simulink model "ModelMy"  (R2023a)
settings: Solver=VariableStepAuto  StartTime=0.0  StopTime=0.01  FixedStep=1E-9  MaxStep=1E-9  RelTol=1e-5
libraries: spsDiodeLib x8, spsSeriesRLCBranchLib x8, spsIdealSwitchLib x4, simulink x3, spsVoltageMeasurementLib x3, spsDCVoltageSourceLib x1, spsGroundLib x1, spsLinearTransformerLib x1, spsMultimeterLib x1, simulink_extras x1, spspowerguiLib x1
settings Model: Creator=kva  LastModifiedBy=User
settings SolverCC: AlgebraicLoopSolver=TrustRegion
settings DataIOCC: ReturnWorkspaceOutputs=off
settings DebuggingCC: UnconnectedInputMsg=warning  UnconnectedOutputMsg=warning  UnconnectedLineMsg=warning  ArithmeticOperatorsInVariantConditions=warning
settings ModelReferenceCC: EnableRefExpFcnMdlSchedulingChecks=on
settings SFSimCC: CustomCodeUndefinedFunction=UseInterfaceOnly

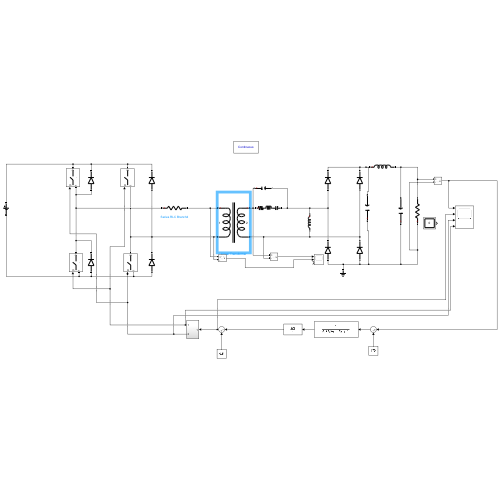
[thumbnail: Simulink's stored preview of the top-level diagram]
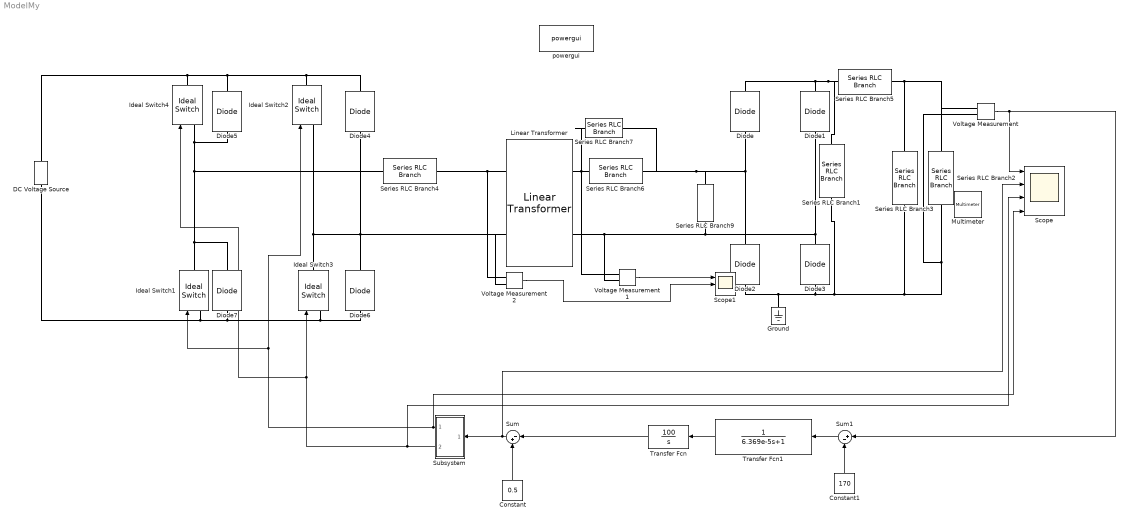
== system ModelMy ==
  Constant : Constant  Value=0.5
  Constant1 : Constant  Value=170
  DC Voltage Source : spsDCVoltageSourceLib/DC Voltage Source  Amplitude=42  Measurements=Voltage
  Diode{,1..7} (8 alike) : spsDiodeLib/Diode  Ron=0.001  Lon=0  Vf=1  IC=0  UseSnubber=0  Rs=inf  Cs=250e-9  Measurements=off
  Ground : spsGroundLib/Ground  LConnTagsString=a
  Ideal Switch{1..4} (4 alike) : spsIdealSwitchLib/Ideal Switch  Ron=0.001  Lon=0  IC=1  Rs=inf  Cs=inf  Measurements=off
  Linear Transformer : spsLinearTransformerLib/Linear Transformer  UNITS=SI  NominalPower=[ 250e6 60 ]  winding1=[42 0 0]  winding2=[170 0 0]  ThreeWindings=off  winding3=[3.15e+05 0.7938 0.084225]  RmLm=[Inf Inf]  Measurements=None  DataType=on
  Multimeter : spsMultimeterLib/Multimeter  L=2  sel=1  yselected={}  Gain=0  OutputType=Complex  PlotAtSimulationStop=off  PhasorSimulation=off
  Scope : Scope  NumInputPorts=4
  Scope1 : Scope  NumInputPorts=3
  Series RLC Branch1 : spsSeriesRLCBranchLib/Series RLC Branch  LConnTagsString=__new0  RConnTagsString=__new0  BranchType=C  Resistance=1  Inductance=1e-3  SetiL0=off  InitialCurrent=0  Capacitance=1e-9  Setx0=off  InitialVoltage=0  Measurements=None
  Series RLC Branch2 : spsSeriesRLCBranchLib/Series RLC Branch  LConnTagsString=__new0  RConnTagsString=__new0  BranchType=R  Resistance=25  Inductance=1e-3  SetiL0=off  InitialCurrent=0  Capacitance=1e-6  Setx0=off  InitialVoltage=0  Measurements=Branch voltage
  Series RLC Branch3 : spsSeriesRLCBranchLib/Series RLC Branch  LConnTagsString=__new0  RConnTagsString=__new0  BranchType=C  Resistance=1  Inductance=1e-3  SetiL0=off  InitialCurrent=0  Capacitance=50e-6  Setx0=off  InitialVoltage=0  Measurements=None
  Series RLC Branch4 : spsSeriesRLCBranchLib/Series RLC Branch  LConnTagsString=__new0  RConnTagsString=__new0  BranchType=R  Resistance=0.01  Inductance=4e-6  SetiL0=off  InitialCurrent=0  Capacitance=154e-9  Setx0=off  InitialVoltage=0  Measurements=None
  Series RLC Branch5 : spsSeriesRLCBranchLib/Series RLC Branch  LConnTagsString=__new0  RConnTagsString=__new0  BranchType=L  Resistance=100  Inductance=100e-6  SetiL0=off  InitialCurrent=0  Capacitance=1e-9  Setx0=off  InitialVoltage=0  Measurements=None
  Series RLC Branch6 : spsSeriesRLCBranchLib/Series RLC Branch  LConnTagsString=__new0  RConnTagsString=__new0  BranchType=RLC  Resistance=0.01  Inductance=4e-6  SetiL0=off  InitialCurrent=0  Capacitance=154e-9  Setx0=off  InitialVoltage=0  Measurements=None
  Series RLC Branch7 : spsSeriesRLCBranchLib/Series RLC Branch  LConnTagsString=__new0  RConnTagsString=__new0  BranchType=C  Resistance=0.01  Inductance=4e-6  SetiL0=off  InitialCurrent=0  Capacitance=1e-9  Setx0=off  InitialVoltage=0  Measurements=None
  Series RLC Branch9 : spsSeriesRLCBranchLib/Series RLC Branch  LConnTagsString=__new0  RConnTagsString=__new0  BranchType=L  Resistance=1  Inductance=30e-6  SetiL0=off  InitialCurrent=0  Capacitance=1e-6  Setx0=off  InitialVoltage=0  Measurements=None
  Subsystem : Subsystem
  Sum : Sum  Inputs=|-+
  Sum1 : Sum  Inputs=|+-
  Transfer Fcn : TransferFcn  Numerator=[100]  Denominator=[1 0]
  Transfer Fcn1 : TransferFcn  Denominator=[6.369e-5 1]
  Voltage Measurement : spsVoltageMeasurementLib/Voltage Measurement  PhasorSimulation=off  OutputType=Complex  PSBequivalent=0
  Voltage Measurement1 : spsVoltageMeasurementLib/Voltage Measurement  PhasorSimulation=off  OutputType=Complex  PSBequivalent=0
  Voltage Measurement2 : spsVoltageMeasurementLib/Voltage Measurement  PhasorSimulation=off  OutputType=Complex  PSBequivalent=0
  powergui : spspowerguiLib/powergui  Priority=1  SimulationMode=Continuous  SampleTime=50e-6  frequency=60  Iterations=50  frequencyindice=0  Pbase=100e6  ErrMax=1e-4  UnitsV=kV  UnitsW=MW  buscounter=0  FunctionMessages=on  echomessages=on  EnableUseOfTLC=on  CurrentSourceSwitches=off  DisableSnubberDevices=off  DisableRonSwitches=off  DisableVfSwitches=on  DisplayEquations=off  AutomaticDiscreteSolvers=off  SolverType=Tustin/Backward Euler (TBE)  Interpol=off  ExternalGateDelay=off  methode=off  Ts=100  x0status=zero  SPID=on  SwTol=0  HookPort=off  NonlinearTolerance=1e-4  nMaxIteration=100  ContinueOnMaxIteration=off  RestoreLinks=warning  ResistiveCurrentMeasurement=off  Frange=[0:2:500]  Ylog=off  Xlog=on  ShowGrid=off  save=off  variable=ZData  structure=ScopeData  ZoomFFT=on  StartTime=0.002  cycles=1  DisplayStyle=4  fundamental=250  FreqAxis=off  MaxFrequency=1000  frequencyindicesteady=1  RmsSteady=1  display=off
  wires:
  Subsystem/1(Out1) -> Scope/4, Ideal Switch1/1, Ideal Switch2/1
  Sum/1 -> Scope/2, Subsystem/1(In1)
  Constant/1 -> Sum/2
  Transfer Fcn1/1 -> Transfer Fcn/1
  Sum1/1 -> Transfer Fcn1/1
  Constant1/1 -> Sum1/2
  Voltage Measurement1/1 -> Scope1/1
  Voltage Measurement2/1 -> Scope1/2
  Subsystem/2(Out2) -> Scope/3, Ideal Switch4/1, Ideal Switch3/1
  Transfer Fcn/1 -> Sum/1
  Voltage Measurement/1 -> Sum1/1, Scope/1
  connections:
  Ideal Switch3/RConn1 -- Diode6/RConn1 -- Diode4/LConn1 -- Voltage Measurement2/LConn2 -- Linear Transformer/LConn2 -- Ideal Switch2/LConn1
  Ideal Switch2/RConn1 -- Diode4/RConn1 -- Diode5/RConn1 -- Ideal Switch4/RConn1 -- DC Voltage Source/RConn1
  Ideal Switch3/LConn1 -- Diode6/LConn1 -- Diode7/LConn1 -- Ideal Switch1/LConn1 -- DC Voltage Source/LConn1
  Diode1/LConn1 -- Diode3/RConn1 -- Series RLC Branch9/RConn1 -- Voltage Measurement1/LConn2 -- Linear Transformer/RConn2
  Series RLC Branch2/LConn1 -- Voltage Measurement/LConn2 -- Series RLC Branch3/LConn1 -- Diode3/LConn1 -- Ground/LConn1 -- Diode2/LConn1 -- Series RLC Branch1/LConn1
  Series RLC Branch3/RConn1 -- Series RLC Branch2/RConn1 -- Voltage Measurement/LConn1 -- Series RLC Branch5/RConn1
  Series RLC Branch5/LConn1 -- Diode1/RConn1 -- Diode/RConn1 -- Series RLC Branch1/RConn1
  Diode/LConn1 -- Series RLC Branch7/RConn1 -- Series RLC Branch6/RConn1 -- Series RLC Branch9/LConn1 -- Diode2/RConn1
  Linear Transformer/LConn1 -- Voltage Measurement2/LConn1 -- Series RLC Branch4/RConn1
  Linear Transformer/RConn1 -- Series RLC Branch7/LConn1 -- Voltage Measurement1/LConn1 -- Series RLC Branch6/LConn1
  Diode7/RConn1 -- Series RLC Branch4/LConn1 -- Diode5/LConn1 -- Ideal Switch4/LConn1 -- Ideal Switch1/RConn1

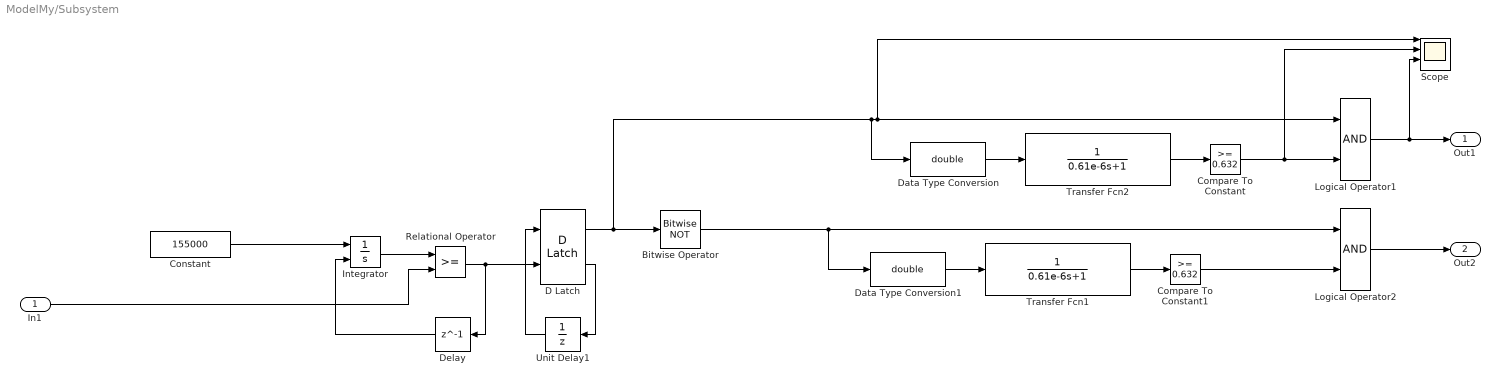
== system ModelMy/Subsystem ==
  In1 : Inport
  Bitwise Operator : simulink/Logic and Bit Operations/Bitwise Operator  logicop=NOT  UseBitMask=off  BitMask=bin2dec('11011001')  BitMaskRealWorld=Stored Integer
  Compare To Constant : simulink/Logic and Bit Operations/Compare To Constant  relop=>=  const=0.632  OutDataTypeStr=boolean
  Compare To Constant1 : simulink/Logic and Bit Operations/Compare To Constant  relop=>=  const=0.632  OutDataTypeStr=boolean
  Constant : Constant  Value=155000
  D Latch : simulink_extras/Flip Flops/D Latch
  Data Type Conversion : DataTypeConversion  OutDataTypeStr=double  SaturateOnIntegerOverflow=off  RndMeth=Floor
  Data Type Conversion1 : DataTypeConversion  OutDataTypeStr=double  SaturateOnIntegerOverflow=off  RndMeth=Floor
  Delay : Delay  DelayLength=1  InitialCondition=0
  Integrator : Integrator  ExternalReset=rising
  Logical Operator1 : Logic  AllPortsSameDT=off  OutDataTypeStr=boolean
  Logical Operator2 : Logic  AllPortsSameDT=off  OutDataTypeStr=boolean
  Relational Operator : RelationalOperator  OutDataTypeStr=boolean  RndMeth=Simplest  InputSameDT=off
  Scope : Scope  NumInputPorts=4
  Transfer Fcn1 : TransferFcn  Denominator=[0.61e-6 1]
  Transfer Fcn2 : TransferFcn  Denominator=[0.61e-6 1]
  Unit Delay1 : UnitDelay  SampleTime=-1  HasFrameUpgradeWarning=on
  Out1 : Outport  VectorParamsAs1DForOutWhenUnconnected=off
  Out2 : Outport  Port=2  VectorParamsAs1DForOutWhenUnconnected=off
  wires:
  Unit Delay1/1 -> D Latch/1
  Integrator/1 -> Relational Operator/1
  D Latch/2 -> Unit Delay1/1
  Constant/1 -> Integrator/1
  Relational Operator/1 -> Delay/1, D Latch/2
  Delay/1 -> Integrator/2
  D Latch/1 -> Data Type Conversion/1, Scope/1, Logical Operator1/1, Bitwise Operator/1
  Compare To Constant/1 -> Scope/2, Logical Operator1/2
  Compare To Constant1/1 -> Logical Operator2/2
  Logical Operator1/1 -> Scope/3, Out1/1
  Logical Operator2/1 -> Out2/1
  In1/1 -> Relational Operator/2
  Data Type Conversion/1 -> Transfer Fcn2/1
  Transfer Fcn2/1 -> Compare To Constant/1
  Data Type Conversion1/1 -> Transfer Fcn1/1
  Transfer Fcn1/1 -> Compare To Constant1/1
  Bitwise Operator/1 -> Data Type Conversion1/1, Logical Operator2/1
